simulink model "Simulink_simulazione1"  (R2021b)
settings: Solver=VariableStepAuto  StartTime=0.0  StopTime=100  RelTol=1e-3
values from neighbouring files (symbols this model uses):
  sys = ss(A, B, C, D)    [Progetto_controllore.m]
undefined symbols (not defined in the file or in its folder): Cc, Gc
settings Model: Creator=Antonio  LastModifiedBy=Antonio

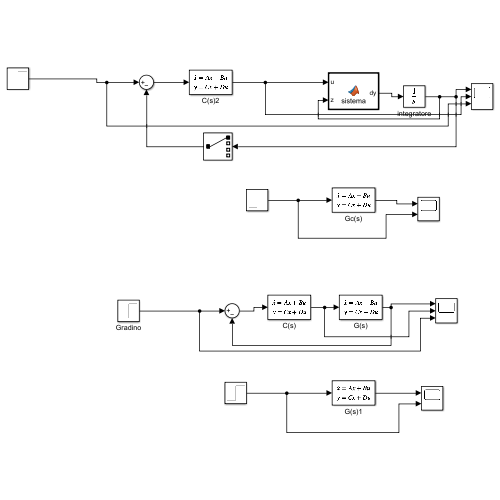
[thumbnail: Simulink's stored preview of the top-level diagram]
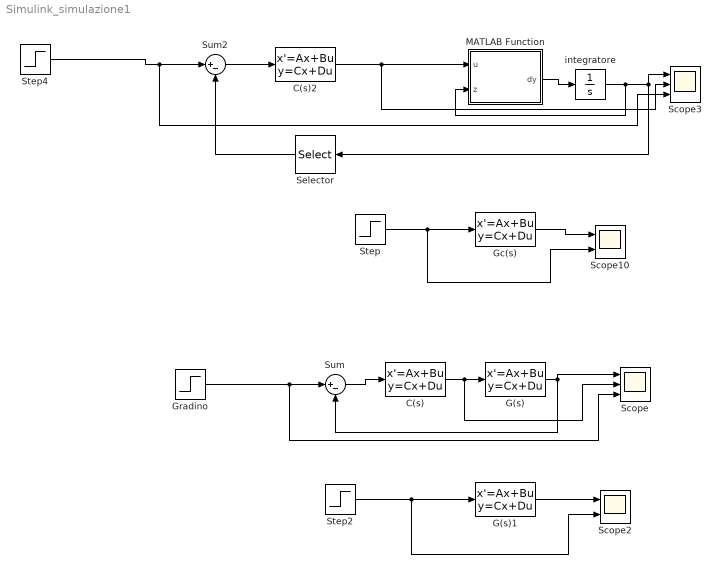
== system Simulink_simulazione1 ==
  C(s) : StateSpace  A=Cc.A  B=Cc.B  C=Cc.C  D=Cc.D  InitialCondition=0
  C(s)2 : StateSpace  A=Cc.A  B=Cc.B  C=Cc.C  D=Cc.D  InitialCondition=0
  G(s) : StateSpace  A=sys.A  B=sys.B  C=sys.C  D=sys.D  InitialCondition=0
  G(s)1 : StateSpace  A=sys.A  B=sys.B  C=sys.C  D=sys.D  InitialCondition=0
  Gc(s) : StateSpace  A=Gc.A  B=Gc.B  C=Gc.C  D=Gc.D  InitialCondition=0
  Gradino : Step  Time=0  SampleTime=0
  MATLAB Function : MATLAB Function  TreatAsAtomicUnit=on
  Scope : Scope  NumInputPorts=3
  Scope10 : Scope  NumInputPorts=2
  Scope2 : Scope  NumInputPorts=2
  Scope3 : Scope  NumInputPorts=3
  Selector : Selector  InputPortWidth=4  IndexOptions=Index vector (dialog)  Indices=[1]  OutputSizes=1
  Step : Step  SampleTime=0
  Step2 : Step  SampleTime=0
  Step4 : Step  SampleTime=0
  Sum : Sum  Inputs=|+-
  Sum2 : Sum  Inputs=|+-
  integratore : Integrator
  wires:
  Step/1 -> Scope10/2, Gc(s)/1
  Gc(s)/1 -> Scope10/1
  G(s)/1 -> Scope/1, Sum/2
  G(s)1/1 -> Scope2/1
  Step2/1 -> Scope2/2, G(s)1/1
  Gradino/1 -> Scope/3, Sum/1
  Sum/1 -> C(s)/1
  C(s)/1 -> Scope/2, G(s)/1
  MATLAB Function/1(dy) -> integratore/1
  integratore/1 -> MATLAB Function/2(z), Selector/1, Scope3/1
  C(s)2/1 -> Scope3/2, MATLAB Function/1(u)
  Step4/1 -> Scope3/3, Sum2/1
  Sum2/1 -> C(s)2/1
  Selector/1 -> Sum2/2

== matlab function Simulink_simulazione1/MATLAB Function ==
  data: u input size=1; z input size=4; dy output size=4
function dy = sistema(u, z)
    %Parametri
    kteta = 143;
    kr = 168;
    b = 1.2;
   % teta = pi/6;
    B = 20;
   % F = -kteta/(2*b); 
   theta_sign = pi/6
    F_sign = -(kteta*sin(theta_sign))/b;
    FL=(F_sign*cos(theta_sign)-B)/sin(theta_sign);
    kzeta = 133;
    M = 580;
    J = 560;
     %stati
    x = z(1);
    v = z(2);
    theta = z(3);
    omega = z(4);
    %Ingressi
    f=u;
    %temp 
    cth = cos(theta); sth=sin(theta); costM=(1/M); costJ=-(1/J);
    %Dinamica
    dx = v;
    dv = costM*(-kzeta*v-cth-FL*sth+B-f*cth);
    dtheta = omega;
    domega =costJ*(kr*omega+kteta*sth+f*b);

   dy =[dx; dv; dtheta; domega];
end
